simulink model "RmtAPP_VD"  (R2016b)
settings: configuration reference "CodeGenConfigSet" (kept outside this file)
values from neighbouring files (symbols this model uses):
  MoFRmtAPP_rLinAPPCURCalMsgA_CUR = Calibration.Parameter    [init_RmtAPP_VD.m]    (also in init_RmtAPP_VD_SIL.m = Simulink.Parameter)
  MoFRmtAPP_rLinAPPCURCalMsgA_CURX = Calibration.Parameter    [init_RmtAPP_VD.m]    (also in init_RmtAPP_VD_SIL.m = Simulink.Parameter)
  RmtAPP_drLinRmp_C = Calibration.Parameter    [init_RmtAPP_VD.m]    (also in init_RmtAPP_VD_SIL.m = Simulink.Parameter)
  RmtAPP_facLowNegPT1_C = Calibration.Parameter    [init_RmtAPP_VD.m]    (also in init_RmtAPP_VD_SIL.m = Simulink.Parameter)
  RmtAPP_facLowPosPT1_C = Calibration.Parameter    [init_RmtAPP_VD.m]    (also in init_RmtAPP_VD_SIL.m = Simulink.Parameter)
  RmtAPP_facMidNegPT1_C = Calibration.Parameter    [init_RmtAPP_VD.m]    (also in init_RmtAPP_VD_SIL.m = Simulink.Parameter)
  RmtAPP_facMidPosPT1_C = Calibration.Parameter    [init_RmtAPP_VD.m]    (also in init_RmtAPP_VD_SIL.m = Simulink.Parameter)
  RmtAPP_facUppNegPT1_C = Calibration.Parameter    [init_RmtAPP_VD.m]    (also in init_RmtAPP_VD_SIL.m = Simulink.Parameter)
  RmtAPP_facUppPosPT1_C = Calibration.Parameter    [init_RmtAPP_VD.m]    (also in init_RmtAPP_VD_SIL.m = Simulink.Parameter)
  RmtAPP_rThrFltLowNeg_C = Calibration.Parameter    [init_RmtAPP_VD.m]    (also in init_RmtAPP_VD_SIL.m = Simulink.Parameter)
  RmtAPP_rThrFltLowPos_C = Calibration.Parameter    [init_RmtAPP_VD.m]    (also in init_RmtAPP_VD_SIL.m = Simulink.Parameter)
  RmtAPP_rThrFltMidNeg_C = Calibration.Parameter    [init_RmtAPP_VD.m]    (also in init_RmtAPP_VD_SIL.m = Simulink.Parameter)
  RmtAPP_rThrFltMidPos_C = Calibration.Parameter    [init_RmtAPP_VD.m]    (also in init_RmtAPP_VD_SIL.m = Simulink.Parameter)
  RmtAPP_swtEnaFlt_C = Calibration.Parameter    [init_RmtAPP_VD.m]    (also in init_RmtAPP_VD_SIL.m = Simulink.Parameter)
  RmtAPP_swtEnaUnJit_C = Calibration.Parameter    [init_RmtAPP_VD.m]    (also in init_RmtAPP_VD_SIL.m = Simulink.Parameter)
  RmtAPP_uJitter_C = Calibration.Parameter    [init_RmtAPP_VD.m]    (also in init_RmtAPP_VD_SIL.m = Simulink.Parameter)
  SigTst_rRmtAPP_C = Calibration.Parameter    [init_RmtAPP_VD.m]    (also in init_RmtAPP_VD_SIL.m = Simulink.Parameter)
  SigTst_swtRmtAPP_C = Calibration.Parameter    [init_RmtAPP_VD.m]    (also in init_RmtAPP_VD_SIL.m = Simulink.Parameter)
undefined symbols (not defined in the file or in its folder): RmtAPP_VD_DT, Switch_conv
libraries: CXLib x5
settings Model: Creator=bianxuyin  LastModifiedBy=bianxuyin
settings ConfigSetRef: SourceLocation=Base Workspace

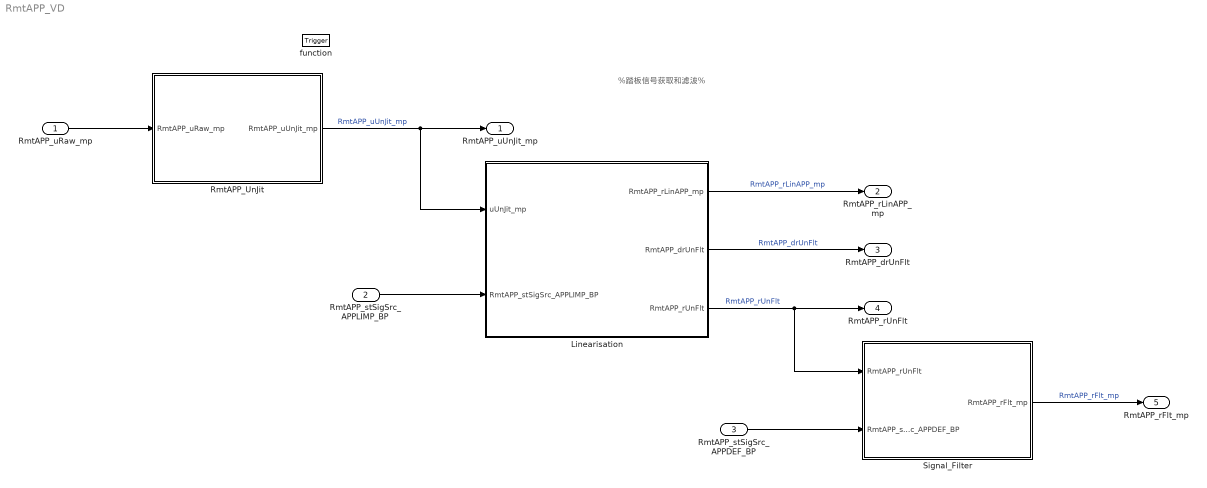
== system RmtAPP_VD ==
  note: %踏板信号获取和滤波%
  RmtAPP_uRaw_mp : Inport  Tag=mv  Description=Remote Acceleration pedal position raw value  OutMin=0  OutMax=5000  OutDataTypeStr=Ad_mv
  RmtAPP_stSigSrc_APPLIMP_BP : Inport  Description=Substitute operation active,remote accelerator pedal sensor value and accelerator pedal sensor increase are limited  Port=2  OutMin=0  OutMax=1  OutDataTypeStr=boolean
  RmtAPP_stSigSrc_APPDEF_BP : Inport  Description=both the sensors are defective. Use the default value  Port=3  OutMin=0  OutMax=1  OutDataTypeStr=boolean
  function : TriggerPort  TriggerType=function-call  VariantControl=Variant
  " Linearisation" : Subsystem
  RmtAPP_UnJit : Subsystem
  Signal_Filter : Subsystem
  RmtAPP_uUnJit_mp : Outport  Tag=mv  Description=Remote Acceleration pedal position unjittered value  OutMin=0  OutMax=5000  OutDataTypeStr=Ad_mv
  RmtAPP_rLinAPP_mp : Outport  Tag=%  Description=Linearisation ratio of remote accelerator pedal  Port=2  OutMin=0  OutMax=100  OutDataTypeStr=Accpedal_rate
  RmtAPP_drUnFlt : Outport  Tag=%/s  Description=Remote Acceleration pedal position gradient of unfilterd value  Port=3  OutMin=-100000  OutMax=100000  OutDataTypeStr=Accpedal_rate_s
  RmtAPP_rUnFlt : Outport  Tag=%  Description=Unfiltered RmtAPP value  Port=4  OutMin=0  OutMax=100  OutDataTypeStr=Accpedal_rate
  RmtAPP_rFlt_mp : Outport  Tag=%  Description=Remote Acceleration pedal position filtered value  Port=5  OutMin=0  OutMax=100  OutDataTypeStr=Accpedal_rate
  wires:
  RmtAPP_UnJit/1(RmtAPP_uUnJit_mp) -> " Linearisation"/1(uUnJit_mp), RmtAPP_uUnJit_mp/1  "RmtAPP_uUnJit_mp"
  " Linearisation"/2(RmtAPP_drUnFlt) -> RmtAPP_drUnFlt/1  "RmtAPP_drUnFlt"
  " Linearisation"/3(RmtAPP_rUnFlt) -> Signal_Filter/1(RmtAPP_rUnFlt), RmtAPP_rUnFlt/1  "RmtAPP_rUnFlt"
  Signal_Filter/1(RmtAPP_rFlt_mp) -> RmtAPP_rFlt_mp/1  "RmtAPP_rFlt_mp"
  RmtAPP_uRaw_mp/1 -> RmtAPP_UnJit/1(RmtAPP_uRaw_mp)
  RmtAPP_stSigSrc_APPLIMP_BP/1 -> " Linearisation"/2(RmtAPP_stSigSrc_APPLIMP_BP)
  " Linearisation"/1(RmtAPP_rLinAPP_mp) -> RmtAPP_rLinAPP_mp/1  "RmtAPP_rLinAPP_mp"
  RmtAPP_stSigSrc_APPDEF_BP/1 -> Signal_Filter/2(RmtAPP_stSigSrc_APPDEF_BP)

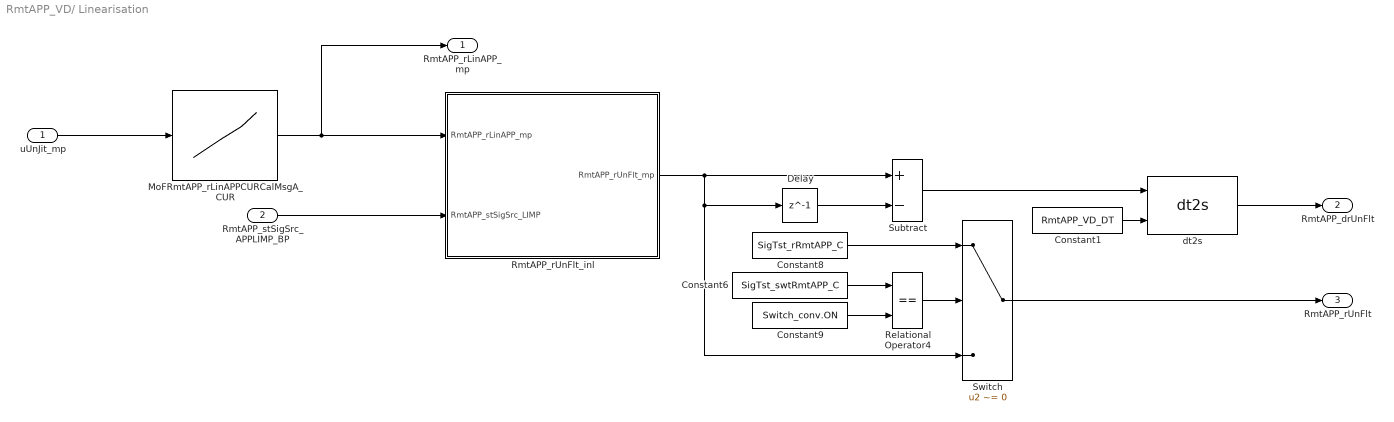
== system RmtAPP_VD/ Linearisation ==
  uUnJit_mp : Inport
  RmtAPP_stSigSrc_APPLIMP_BP : Inport  Tag=-  Description=Substitute operation active, accelerator pedal sensor value and accelerator pedal sensor increase are limited  Port=2  OutMin=0  OutMax=1  OutDataTypeStr=boolean
  Constant1 : Constant  Value=RmtAPP_VD_DT  OutDataTypeStr=Inherit: Inherit via back propagation
  Constant6 : Constant  Value=SigTst_swtRmtAPP_C
  Constant8 : Constant  Value=SigTst_rRmtAPP_C
  Constant9 : Constant  Value=Switch_conv.ON  OutDataTypeStr=Inherit: Inherit via back propagation
  Delay : Delay  DelayLength=1  InitialCondition=0
  MoFRmtAPP_rLinAPPCURCalMsgA_CUR : Lookup_n-D  NumberOfTableDimensions=1  BreakpointsForDimension1=MoFRmtAPP_rLinAPPCURCalMsgA_CURX  IndexSearchMethod=Linear search  BeginIndexSearchUsingPreviousIndexResult=on  UseOneInputPortForAllInputData=on  Table=MoFRmtAPP_rLinAPPCURCalMsgA_CUR  ExtrapMethod=Clip  UseLastTableValue=on  InternalRulePriority=Speed  OutDataTypeStr=Inherit: Inherit via back propagation  SaturateOnIntegerOverflow=on
  Relational Operator4 : RelationalOperator  Operator===  OutDataTypeStr=boolean  RndMeth=Simplest  InputSameDT=on
  RmtAPP_rUnFlt_inl : Subsystem
  Subtract : Sum  Inputs=+-  OutDataTypeStr=Inherit: Inherit via back propagation  InputSameDT=on
  Switch : Switch  Criteria=u2 ~= 0  InputSameDT=on
  dt2s : CXLib/dt2s
  RmtAPP_rLinAPP_mp : Outport  Tag=%%  Description=Linearisation ratio of accelerator pedal
  RmtAPP_drUnFlt : Outport  Tag=%%  Description=Acceleration pedal position gradient of unfilterd value  Port=2
  RmtAPP_rUnFlt : Outport  Tag=%%  Description=Unfiltered APP value  Port=3
  wires:
  uUnJit_mp/1 -> MoFRmtAPP_rLinAPPCURCalMsgA_CUR/1
  MoFRmtAPP_rLinAPPCURCalMsgA_CUR/1 -> RmtAPP_rLinAPP_mp/1, RmtAPP_rUnFlt_inl/1(RmtAPP_rLinAPP_mp)
  RmtAPP_stSigSrc_APPLIMP_BP/1 -> RmtAPP_rUnFlt_inl/2(RmtAPP_stSigSrc_LIMP)
  Relational Operator4/1 -> Switch/2
  Constant6/1 -> Relational Operator4/1
  Constant9/1 -> Relational Operator4/2
  Constant8/1 -> Switch/1
  RmtAPP_rUnFlt_inl/1(RmtAPP_rUnFlt_mp) -> Switch/3, Delay/1, Subtract/1
  Delay/1 -> Subtract/2
  Subtract/1 -> dt2s/1
  Constant1/1 -> dt2s/2
  dt2s/1 -> RmtAPP_drUnFlt/1
  Switch/1 -> RmtAPP_rUnFlt/1

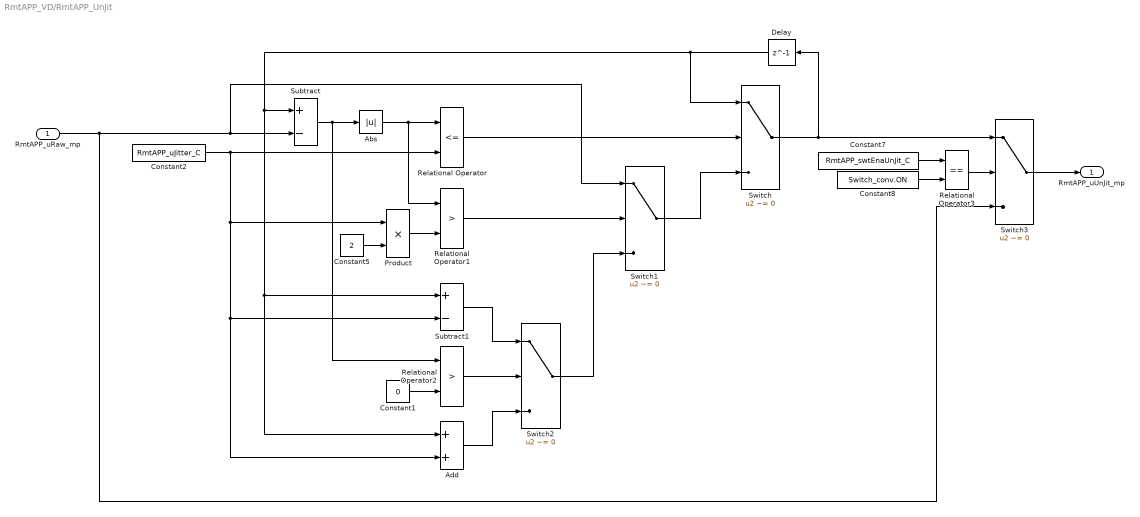
== system RmtAPP_VD/RmtAPP_UnJit ==
  RmtAPP_uRaw_mp : Inport
  Abs : Abs  OutDataTypeStr=Inherit: Inherit via back propagation
  Add : Sum
  Constant1 : Constant  Value=0  OutDataTypeStr=Inherit: Inherit via back propagation
  Constant2 : Constant  Value=RmtAPP_uJitter_C
  Constant5 : Constant  Value=2  OutDataTypeStr=Inherit: Inherit via back propagation
  Constant7 : Constant  Value=RmtAPP_swtEnaUnJit_C
  Constant8 : Constant  Value=Switch_conv.ON  OutDataTypeStr=Inherit: Inherit via back propagation
  Delay : Delay  DelayLength=1  InitialCondition=0
  Product : Product  OutDataTypeStr=Inherit: Same as first input
  Relational Operator : RelationalOperator  Operator=<=  OutDataTypeStr=boolean  RndMeth=Simplest
  Relational Operator1 : RelationalOperator  Operator=>  OutDataTypeStr=boolean  RndMeth=Simplest
  Relational Operator2 : RelationalOperator  Operator=>  OutDataTypeStr=boolean  RndMeth=Simplest
  Relational Operator3 : RelationalOperator  Operator===  OutDataTypeStr=boolean  RndMeth=Simplest  InputSameDT=on
  Subtract : Sum  Inputs=+-
  Subtract1 : Sum  Inputs=+-
  Switch{,1..3} (4 alike) : Switch  Criteria=u2 ~= 0
  RmtAPP_uUnJit_mp : Outport
  wires:
  RmtAPP_uRaw_mp/1 -> Switch3/3, Switch1/1, Subtract/2
  Subtract/1 -> Abs/1, Relational Operator2/1
  Abs/1 -> Relational Operator1/1, Relational Operator/1
  Product/1 -> Relational Operator1/2
  Constant5/1 -> Product/2
  Constant2/1 -> Relational Operator/2, Add/2, Subtract1/2, Product/1
  Switch/1 -> Switch3/1, Delay/1
  Relational Operator1/1 -> Switch1/2
  Switch1/1 -> Switch/3
  Relational Operator/1 -> Switch/2
  Constant1/1 -> Relational Operator2/2
  Delay/1 -> Add/1, Subtract1/1, Subtract/1, Switch/1
  Relational Operator2/1 -> Switch2/2
  Switch2/1 -> Switch1/3
  Subtract1/1 -> Switch2/1
  Add/1 -> Switch2/3
  Constant7/1 -> Relational Operator3/1
  Constant8/1 -> Relational Operator3/2
  Relational Operator3/1 -> Switch3/2
  Switch3/1 -> RmtAPP_uUnJit_mp/1

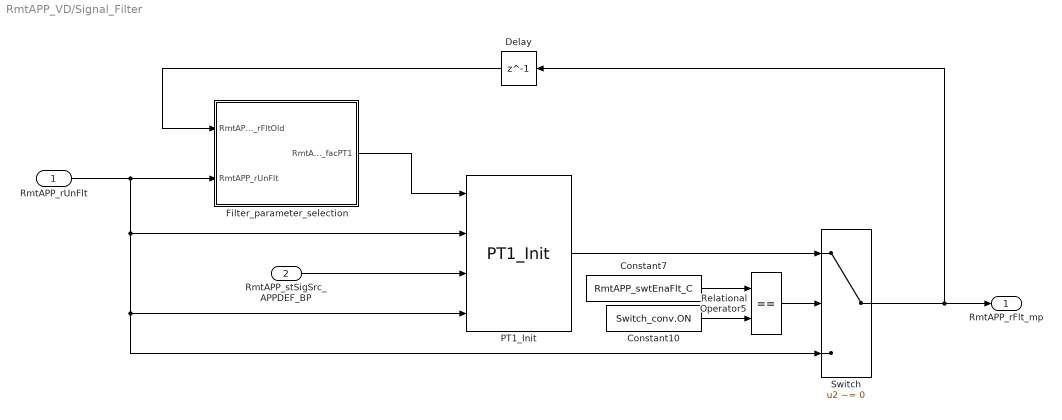
== system RmtAPP_VD/Signal_Filter ==
  RmtAPP_rUnFlt : Inport
  RmtAPP_stSigSrc_APPDEF_BP : Inport  Tag=-  Description=both the sensors are defective. Use the default value  Port=2  OutMin=0  OutMax=1  OutDataTypeStr=boolean
  Constant10 : Constant  Value=Switch_conv.ON  OutDataTypeStr=Inherit: Inherit via back propagation
  Constant7 : Constant  Value=RmtAPP_swtEnaFlt_C
  Delay : Delay  DelayLength=1  InitialCondition=0
  Filter_parameter_selection : Subsystem  TreatAsAtomicUnit=on
  PT1_Init : CXLib/PT1_Init
  Relational Operator5 : RelationalOperator  Operator===  OutDataTypeStr=boolean  RndMeth=Simplest  InputSameDT=on
  Switch : Switch  Criteria=u2 ~= 0
  RmtAPP_rFlt_mp : Outport  Tag=%%  Description=Acceleration pedal position filtered value
  wires:
  RmtAPP_rUnFlt/1 -> Switch/3, PT1_Init/4, PT1_Init/2, Filter_parameter_selection/2(RmtAPP_rUnFlt)
  Filter_parameter_selection/1(RmtAPP_facPT1) -> PT1_Init/1
  RmtAPP_stSigSrc_APPDEF_BP/1 -> PT1_Init/3
  Relational Operator5/1 -> Switch/2
  Constant10/1 -> Relational Operator5/2
  Constant7/1 -> Relational Operator5/1
  PT1_Init/1 -> Switch/1
  Switch/1 -> Delay/1, RmtAPP_rFlt_mp/1
  Delay/1 -> Filter_parameter_selection/1(RmtAPP_rFltOld)

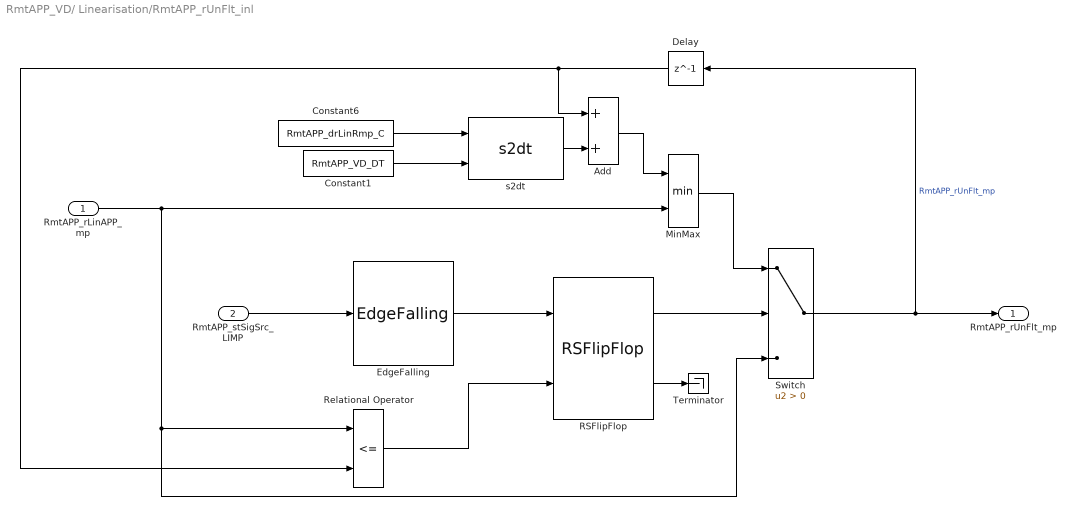
== system RmtAPP_VD/ Linearisation/RmtAPP_rUnFlt_inl ==
  RmtAPP_rLinAPP_mp : Inport
  RmtAPP_stSigSrc_LIMP : Inport  Port=2
  Add : Sum  InputSameDT=on
  Constant1 : Constant  Value=RmtAPP_VD_DT  OutDataTypeStr=Inherit: Inherit via back propagation
  Constant6 : Constant  Value=RmtAPP_drLinRmp_C
  Delay : Delay  DelayLength=1  InitialCondition=0
  EdgeFalling : CXLib/EdgeFalling
  MinMax : MinMax  Inputs=2
  RSFlipFlop : CXLib/RSFlipFlop
  Relational Operator : RelationalOperator  Operator=<=  OutDataTypeStr=boolean  RndMeth=Simplest  InputSameDT=on
  Switch : Switch  Criteria=u2 > Threshold
  Terminator : Terminator
  s2dt : CXLib/s2dt
  RmtAPP_rUnFlt_mp : Outport  Tag=mv  Description=Remote Acceleration pedal position unjittered value
  wires:
  RmtAPP_stSigSrc_LIMP/1 -> EdgeFalling/1
  Constant1/1 -> s2dt/2
  Constant6/1 -> s2dt/1
  s2dt/1 -> Add/2
  RmtAPP_rLinAPP_mp/1 -> Switch/3, Relational Operator/1, MinMax/2
  Add/1 -> MinMax/1
  EdgeFalling/1 -> RSFlipFlop/1
  RSFlipFlop/1 -> Switch/2
  MinMax/1 -> Switch/1
  Switch/1 -> Delay/1, RmtAPP_rUnFlt_mp/1  "RmtAPP_rUnFlt_mp"
  Delay/1 -> Add/1, Relational Operator/2
  RSFlipFlop/2 -> Terminator/1
  Relational Operator/1 -> RSFlipFlop/2

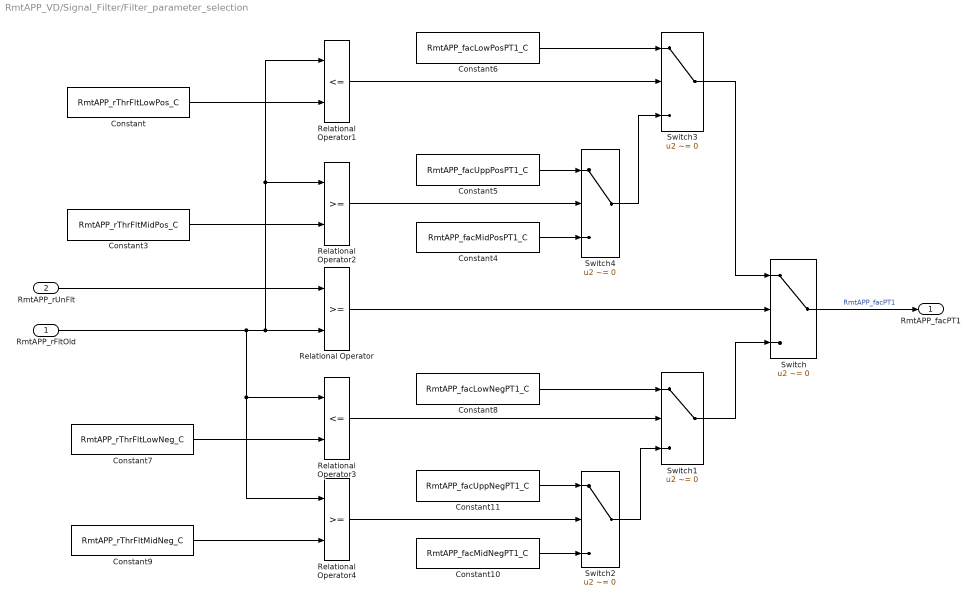
== system RmtAPP_VD/Signal_Filter/Filter_parameter_selection ==
  RmtAPP_rFltOld : Inport
  RmtAPP_rUnFlt : Inport  Port=2
  Constant : Constant  Value=RmtAPP_rThrFltLowPos_C
  Constant10 : Constant  Value=RmtAPP_facMidNegPT1_C
  Constant11 : Constant  Value=RmtAPP_facUppNegPT1_C
  Constant3 : Constant  Value=RmtAPP_rThrFltMidPos_C
  Constant4 : Constant  Value=RmtAPP_facMidPosPT1_C
  Constant5 : Constant  Value=RmtAPP_facUppPosPT1_C
  Constant6 : Constant  Value=RmtAPP_facLowPosPT1_C
  Constant7 : Constant  Value=RmtAPP_rThrFltLowNeg_C
  Constant8 : Constant  Value=RmtAPP_facLowNegPT1_C
  Constant9 : Constant  Value=RmtAPP_rThrFltMidNeg_C
  Relational Operator : RelationalOperator  OutDataTypeStr=boolean  RndMeth=Nearest
  Relational Operator1 : RelationalOperator  Operator=<=  OutDataTypeStr=boolean  RndMeth=Nearest
  Relational Operator2 : RelationalOperator  OutDataTypeStr=boolean  RndMeth=Nearest
  Relational Operator3 : RelationalOperator  Operator=<=  OutDataTypeStr=boolean  RndMeth=Nearest
  Relational Operator4 : RelationalOperator  OutDataTypeStr=boolean  RndMeth=Nearest
  Switch{,1..4} (5 alike) : Switch  Criteria=u2 ~= 0  Threshold=1  InputSameDT=on
  RmtAPP_facPT1 : Outport
  wires:
  Constant/1 -> Relational Operator1/2
  Constant3/1 -> Relational Operator2/2
  Constant7/1 -> Relational Operator3/2
  Constant9/1 -> Relational Operator4/2
  Relational Operator/1 -> Switch/2
  Constant8/1 -> Switch1/1
  Constant11/1 -> Switch2/1
  Constant10/1 -> Switch2/3
  Relational Operator4/1 -> Switch2/2
  Switch2/1 -> Switch1/3
  Relational Operator3/1 -> Switch1/2
  Constant6/1 -> Switch3/1
  Switch4/1 -> Switch3/3
  Constant5/1 -> Switch4/1
  Constant4/1 -> Switch4/3
  Relational Operator2/1 -> Switch4/2
  Switch3/1 -> Switch/1
  Relational Operator1/1 -> Switch3/2
  RmtAPP_rFltOld/1 -> Relational Operator2/1, Relational Operator1/1, Relational Operator/2, Relational Operator4/1, Relational Operator3/1
  RmtAPP_rUnFlt/1 -> Relational Operator/1
  Switch1/1 -> Switch/3
  Switch/1 -> RmtAPP_facPT1/1  "RmtAPP_facPT1"
